simulink model "LQRsim"  (R2021b)
settings: Solver=VariableStepAuto  StartTime=0.0  StopTime=5  RelTol=1e-3
values from neighbouring files (symbols this model uses):
  d0 = 14    [LQRsetup.m]    (also in PIDsetup.m; datasheet.m = 0.01228; setup.m = 0.01228)
  deltaeq = 7    [LQRsetup.m]
  K = 100    [ElecTFanalysis.m]    (also in LQRgen.m = lqr(A, B, Q , R); LQRsetup.m = lqi(sys, Q, R); LQRval.mat = [1 3.39364810121 0.758423717417])
  mG = gc(1)    [LQRsetup.m]    (also in PIDsetup.m)
  qG = gc(2)    [LQRsetup.m]    (also in PIDsetup.m)
  start = d0    (= 14)    [LQRsetup.m]    (also in PIDsetup.m = 10.5)
libraries: MAGLEV_components x2, spsFirstOrderFilterLib x1
settings Model: Creator=dfigu  LastModifiedBy=dfigu

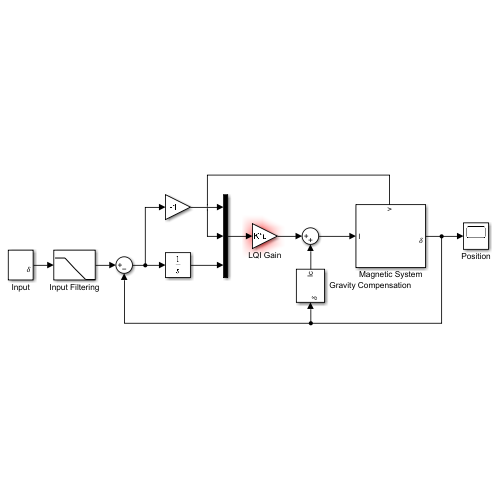
[thumbnail: Simulink's stored preview of the top-level diagram]
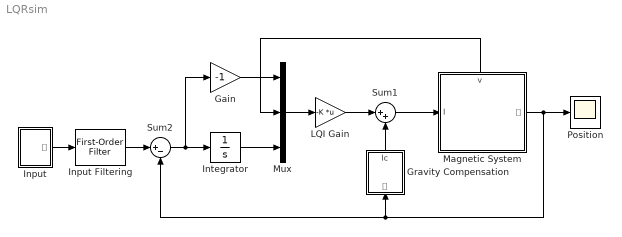
== system LQRsim ==
  Gain : Gain  Gain=-1
  Gravity Compensation : Subsystem
  Input : Subsystem
  Input Filtering : spsFirstOrderFilterLib/First-Order Filter  FilterType=Lowpass  Tc=0.01  Ts=0  Initialize=on  Vac_Init=[0, 0, 60]  Vdc_Init=d0  PlotResponse=off  FreqRange="[0,  200,  1]"
  Integrator : Integrator
  LQI Gain : Gain  Gain=-K  Multiplication=Matrix(K*u)
  Magnetic System : Subsystem
      settings: PortSchema="{\"entries\":[{\"content\":{\"sides\":[{\"content\":{\"connectorIds\":[\"In1\"]},\"type\":\"ConnectorPlacement.EquallySpacedRectSide\",\"uuid\":\"11c028e3-2450-44cd-a965-7c94b7d6c677\"},{\"content\":{\"connectorIds\":[\"Out1\"],\"side\":\"RIGHT\"},\"type\":\"ConnectorPlacement.EquallySpacedRectSide\",\"uuid\":\"426461b2-46d8-43cd-b908-5fc589a9717c\"},{\"content\":{\"connectorIds\":[\"Out2\"],\"side\":\"TOP\"},\"type\":\"ConnectorPlacement.EquallySpacedRectSide\",\"uuid\":\"67341ad5-b114-4454-87f9-8b536917aa78\"}]},\"type\":\"ConnectorPlacement.EquallySpacedConnector\",\"uuid\":\"6dec0cc7-4a6d-4080-a30f-cd6ad671a8da\"}],\"packageUris\":[\"http://schema.mathworks.com/mf0/Connector/R2020b\"],\"version\":\"1.0\"}"
  Mux : Mux  Inputs=3
  Position : Scope
  Sum1 : Sum  Inputs=|++
  Sum2 : Sum  Inputs=|+-
  wires:
  Gravity Compensation/1(Ic) -> Sum1/2
  Sum1/1 -> Magnetic System/1(I)
  LQI Gain/1 -> Sum1/1
  Sum2/1 -> Gain/1, Integrator/1
  Mux/1 -> LQI Gain/1
  Integrator/1 -> Mux/3
  Magnetic System/1(𝛿) -> Position/1, Sum2/2, Gravity Compensation/1(𝛿)
  Input/1(𝛿) -> Input Filtering/1
  Gain/1 -> Mux/1
  Input Filtering/1 -> Sum2/1
  Magnetic System/2(v) -> Mux/2

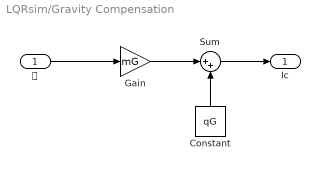
== system LQRsim/Gravity Compensation ==
  𝛿 : Inport
  Constant : Constant  Value=qG
  Gain : Gain  Gain=mG
  Sum : Sum  Inputs=|++
  Ic : Outport
  wires:
  Gain/1 -> Sum/1
  Sum/1 -> Ic/1
  Constant/1 -> Sum/2
  𝛿/1 -> Gain/1

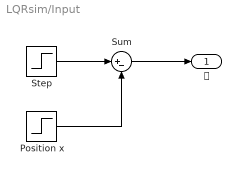
== system LQRsim/Input ==
  Position x : Step  After=deltaeq  SampleTime=0
  Step : Step  Time=0  Before=d0  After=start  SampleTime=0
  Sum : Sum  Inputs=|+-
  𝛿 : Outport
  wires:
  Step/1 -> Sum/1
  Sum/1 -> 𝛿/1
  Position x/1 -> Sum/2

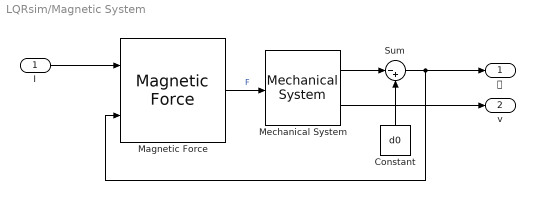
== system LQRsim/Magnetic System ==
  I : Inport
  Constant : Constant  Value=d0
  Magnetic Force : MAGLEV_components/Magnetic Force
      link override 2-D Lookup Table: InterpMethod=Cubic spline  ExtrapMethod=Linear  DiagnosticForOutOfRangeInput=Warning
  Mechanical System : MAGLEV_components/Mechanical System
      link override "Integrator, Second-Order": ICX=0
  Sum : Sum  Inputs=|-+
  𝛿 : Outport
  v : Outport  Port=2
  wires:
  Mechanical System/1 -> Sum/1
  Magnetic Force/1 -> Mechanical System/1  "F"
  Constant/1 -> Sum/2
  I/1 -> Magnetic Force/1
  Mechanical System/2 -> v/1
  Sum/1 -> Magnetic Force/2, 𝛿/1
